simulink model "PF_implementacion_modeloL"  (R2023a)
settings: Solver=VariableStepAuto  StartTime=0.0  StopTime=10.0  RelTol=1e-3
settings Model: Creator=ja616  LastModifiedBy=ja616

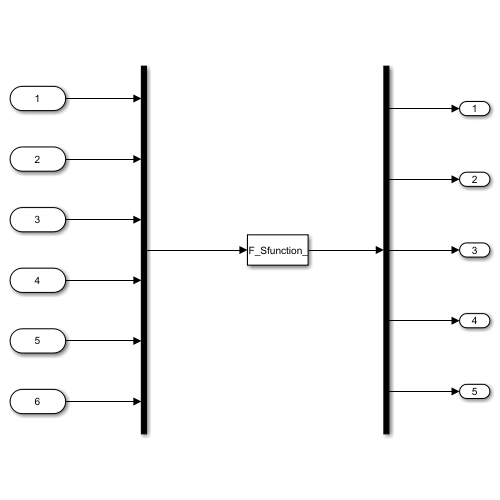
[thumbnail: Simulink's stored preview of the top-level diagram]
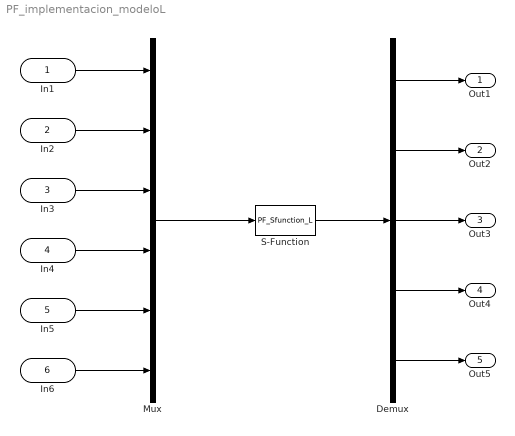
== system PF_implementacion_modeloL ==
  In1 : Inport
  In2 : Inport  Port=2
  In3 : Inport  Port=3
  In4 : Inport  Port=4
  In5 : Inport  Port=5
  In6 : Inport  Port=6
  Demux : Demux  Outputs=5
  Mux : Mux  Inputs=6
  S-Function : S-Function  FunctionName=PF_Sfunction_L  SFunctionDeploymentMode=off  EnableBusSupport=off
  Out1 : Outport
  Out2 : Outport  Port=2
  Out3 : Outport  Port=3
  Out4 : Outport  Port=4
  Out5 : Outport  Port=5
  wires:
  In1/1 -> Mux/1
  In2/1 -> Mux/2
  In3/1 -> Mux/3
  In4/1 -> Mux/4
  In5/1 -> Mux/5
  In6/1 -> Mux/6
  Mux/1 -> S-Function/1
  S-Function/1 -> Demux/1
  Demux/1 -> Out1/1
  Demux/2 -> Out2/1
  Demux/3 -> Out3/1
  Demux/4 -> Out4/1
  Demux/5 -> Out5/1
